simulink model "look1up"  (R2017a)
settings: Solver=FixedStepAuto  StartTime=0.0  StopTime=0.004  RelTol=1e-3
undefined symbols (not defined in the file or in its folder): High
libraries: dspswit3 x2
settings Model: Creator=User  LastModifiedBy=User

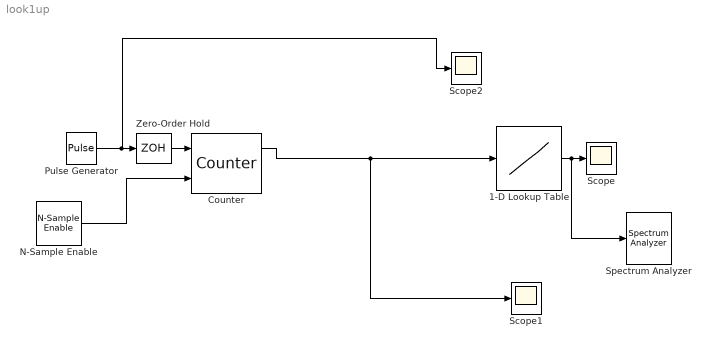
== system look1up ==
  1-D Lookup Table : Lookup_n-D  NumberOfTableDimensions=1  BreakpointsForDimension1=linspace(0,10,10)  Table=sin(linspace(0,2*pi,10))  InternalRulePriority=Speed  RndMeth=Simplest  InputSameDT=on
  Counter : dspswit3/Counter  Direction=Up  CountEvent=Rising edge  CounterSize=User defined  MaxCount=10  InitialCount=0  Output=Count and Hit  HitValue=32  ResetInput=on  SamplesPerFrame=1  Ts=1  CntDtype=double  HitDtype=Logical
  N-Sample Enable : dspswit3/N-Sample Enable  N=10  ActiveLevel=High (1)  reset=off  TriggerType=Rising edge  Ts=1  DataType=Logical
      settings: SourceProductName=DSP System Toolbox  SourceProductBaseCode=DS
  Pulse Generator : DiscretePulseGenerator  PulseType=Time based  Period=1e-5  SampleTime=100
  Scope : Scope
  Scope1 : Scope
  Scope2 : Scope
  Spectrum Analyzer : SpectrumAnalyzer
  Zero-Order Hold : ZeroOrderHold  SampleTime=-1
  wires:
  N-Sample Enable/1 -> Counter/2
  1-D Lookup Table/1 -> Spectrum Analyzer/1, Scope/1
  Counter/1 -> 1-D Lookup Table/1, Scope1/1
  Pulse Generator/1 -> Scope2/1, Zero-Order Hold/1
  Zero-Order Hold/1 -> Counter/1
